simulink model "generator_simulink"  (R2022a)
settings: Solver=VariableStepAuto  StartTime=0.1  StopTime=90  FixedStep=sample_time/10  RelTol=1e-3
values from neighbouring files (symbols this model uses):
  B_eq = rotor.B + generator.B/gearbox.ratio^2    [parameters.m]
  G_noR = Yq*Gc    [generator_m.m]
  Gc = 1/(1 + s*tau_c)    [generator_m.m]    (also in generator_test.m)
  I_eq = rotor.I/gearbox.ratio^2 + generator.I    [main.m]    (also in parameters.m = rotor.I + generator.I/gearbox.ratio^2)
  Iq_ref = 12e3    (= 12000)    [generator_m.m]    (also in generator_test.m = 5000)
  Mr = 1e5    (= 100000)    [generator_m.m]    (also in generator_test.m)
  omega_r_ref = 1    [generator_m.m]    (also in generator_test.m)
  Riq = kiq_p + 1/s*kiq_i + s*kiq_d    [generator_m.m]    (also in generator_test.m)
  Riq_den = Riq.den{1}    [generator_m.m]
  Riq_num = Riq.num{1}    [generator_m.m]
  Romega = komega_p + 1/s*komega_i + s*komega_d    [generator_test.m]
  Yiq = (B+s*I)/(L*I*s^2+(R*I+L*B)*s+R*B+1.5*(p*Lambda)^2)    [generator_test.m]
  Yq = (B + s*I)/(1.5*(p*Lambda)^2*(1 + 2/3*(R + s*L)*(B + s*I)    /(p*Lambda)^2))    [generator_m.m]
undefined symbols (not defined in the file or in its folder): gearbox, generator, omega_r, R_omega_den, R_omega_num, rotor
settings Model: Creator=Niccolò  LastModifiedBy=Niccolò

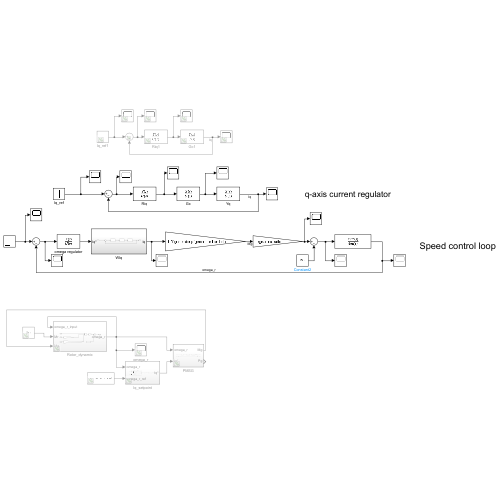
[thumbnail: Simulink's stored preview of the top-level diagram]
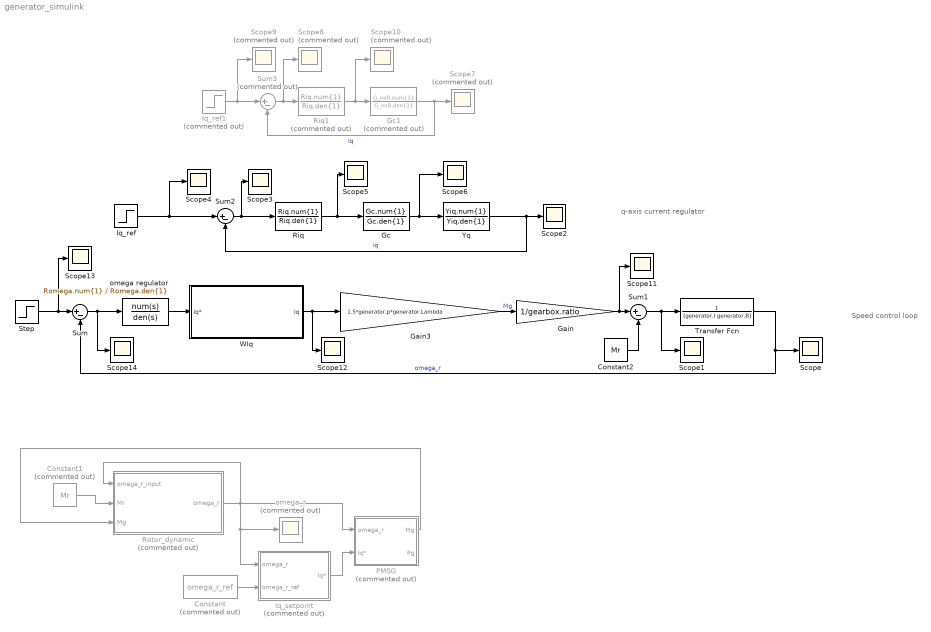
== system generator_simulink ==
  note: Speed control loop
  note: q-axis current regulator
  Constant : Constant  Commented=on  Value=omega_r_ref
  Constant1 : Constant  Commented=on  Value=Mr
  Constant2 : Constant  Value=Mr
  Gain : Gain  Gain=1/gearbox.ratio
  Gain3 : Gain  Gain=1.5*generator.p*generator.Lambda
  Gc : TransferFcn  Numerator=Gc.num{1}  Denominator=Gc.den{1}
  Gc1 : TransferFcn  Commented=on  Numerator=G_noR.num{1}  Denominator=G_noR.den{1}
  Iq_ref : Step  After=Iq_ref  SampleTime=0
  Iq_ref1 : Step  Commented=on  After=Iq_ref  SampleTime=0
  Iq_setpoint : Subsystem  Commented=on
  PMSG : Subsystem  Commented=on
  Riq : TransferFcn  Numerator=Riq.num{1}  Denominator=Riq.den{1}
  Riq1 : TransferFcn  Commented=on  Numerator=Riq.num{1}  Denominator=Riq.den{1}
  Rotor_dynamic : Subsystem  Commented=on
  Scope{,1..6,11..14} (11 alike) : Scope
  Scope{7..10} (4 alike) : Scope  Commented=on
  Step : Step  After=omega_r_ref  SampleTime=0
  Sum : Sum  Inputs=|+-
  Sum1 : Sum  Inputs=|+-
  Sum2 : Sum  Inputs=|+-
  Sum3 : Sum  Commented=on  Inputs=|+-
  Transfer Fcn : TransferFcn  Denominator=[generator.I generator.B]
  WIq : Subsystem
  Yq : TransferFcn  Numerator=Yiq.num{1}  Denominator=Yiq.den{1}
  omega regulator : TransferFcn  Numerator=Romega.num{1}  Denominator=Romega.den{1}
  omega_r : Scope  Commented=on
  wires:
  PMSG/1(Mg) -> Rotor_dynamic/3(Mg)
  Iq_setpoint/1(Iq*) -> PMSG/2(Iq*)
  Rotor_dynamic/1(omega_r) -> Iq_setpoint/1(omega_r), omega_r/1, PMSG/1(omega_r), Rotor_dynamic/1(omega_r_input)
  Constant/1 -> Iq_setpoint/2(omega_r_ref)
  Constant1/1 -> Rotor_dynamic/2(Mr)
  Gain3/1 -> Gain/1  "Mg"
  WIq/1(Iq) -> Scope12/1, Gain3/1
  Sum/1 -> Scope14/1, omega regulator/1
  Sum1/1 -> Scope1/1, Transfer Fcn/1
  Transfer Fcn/1 -> Scope/1, Sum/2  "omega_r"
  Constant2/1 -> Sum1/2
  Step/1 -> Scope13/1, Sum/1
  Riq/1 -> Scope5/1, Gc/1
  Gc/1 -> Scope6/1, Yq/1
  Sum2/1 -> Scope3/1, Riq/1
  Iq_ref/1 -> Scope4/1, Sum2/1
  Yq/1 -> Scope2/1, Sum2/2  "Iq"
  Riq1/1 -> Gc1/1, Scope10/1
  Gc1/1 -> Sum3/2, Scope7/1  "Iq"
  Sum3/1 -> Scope8/1, Riq1/1
  Iq_ref1/1 -> Scope9/1, Sum3/1
  omega regulator/1 -> WIq/1(Iq*)
  Gain/1 -> Scope11/1, Sum1/1

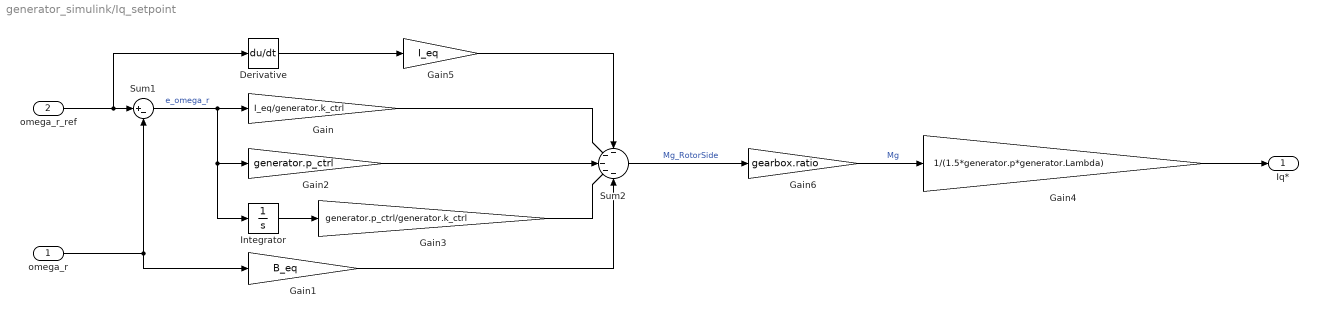
== system generator_simulink/Iq_setpoint ==
  omega_r : Inport
  omega_r_ref : Inport  Port=2
  Derivative : Derivative
  Gain : Gain  Gain=I_eq/generator.k_ctrl
  Gain1 : Gain  Gain=B_eq
  Gain2 : Gain  Gain=generator.p_ctrl
  Gain3 : Gain  Gain=generator.p_ctrl/generator.k_ctrl
  Gain4 : Gain  Gain=1/(1.5*generator.p*generator.Lambda)
  Gain5 : Gain  Gain=I_eq
  Gain6 : Gain  Gain=gearbox.ratio
  Integrator : Integrator
  Sum1 : Sum  Inputs=|+-
  Sum2 : Sum  Inputs=-----
  Iq* : Outport
  wires:
  Gain/1 -> Sum2/2
  Sum1/1 -> Integrator/1, Gain2/1, Gain/1  "e_omega_r"
  Gain1/1 -> Sum2/5
  Gain4/1 -> Iq*/1
  omega_r_ref/1 -> Derivative/1, Sum1/1
  omega_r/1 -> Gain1/1, Sum1/2
  Integrator/1 -> Gain3/1
  Gain3/1 -> Sum2/4
  Gain2/1 -> Sum2/3
  Sum2/1 -> Gain6/1  "Mg_RotorSide"
  Gain5/1 -> Sum2/1
  Gain6/1 -> Gain4/1  "Mg"
  Derivative/1 -> Gain5/1

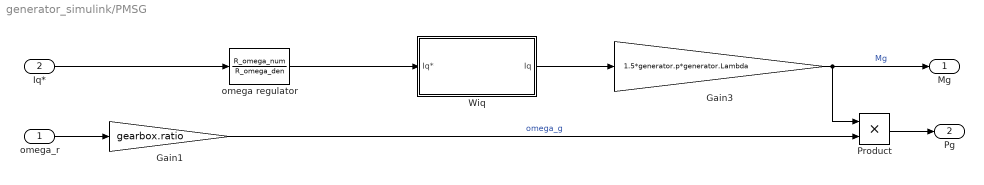
== system generator_simulink/PMSG ==
  omega_r : Inport
  Iq* : Inport  Port=2
  Gain1 : Gain  Gain=gearbox.ratio
  Gain3 : Gain  Gain=1.5*generator.p*generator.Lambda
  Product : Product
  Wiq : Subsystem
  omega regulator : TransferFcn  Numerator=R_omega_num  Denominator=R_omega_den
  Mg : Outport
  Pg : Outport  Port=2
  wires:
  omega_r/1 -> Gain1/1
  Gain3/1 -> Product/1, Mg/1  "Mg"
  Gain1/1 -> Product/2  "omega_g"
  Product/1 -> Pg/1
  Iq*/1 -> omega regulator/1
  Wiq/1(Iq) -> Gain3/1
  omega regulator/1 -> Wiq/1(Iq*)

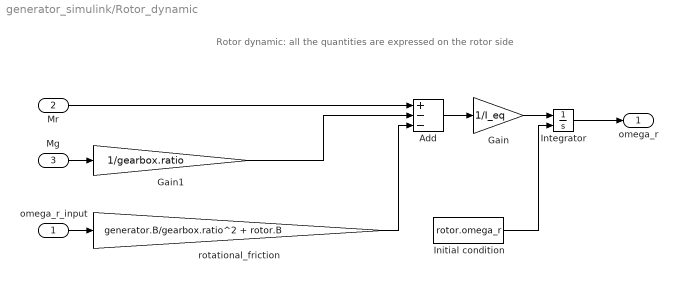
== system generator_simulink/Rotor_dynamic ==
  note: Rotor dynamic: all the quantities are expressed on the rotor side
  omega_r_input : Inport
  Mr : Inport  Port=2
  Mg : Inport  Port=3
  Add : Sum  Inputs=+--
  Gain : Gain  Gain=1/I_eq
  Gain1 : Gain  Gain=1/gearbox.ratio
  Initial condition : Constant  Value=rotor.omega_r
  Integrator : Integrator  InitialConditionSource=external  InitialCondition=omega_r
  rotational_friction : Gain  Gain=generator.B/gearbox.ratio^2 + rotor.B
  omega_r : Outport
  wires:
  Add/1 -> Gain/1
  Gain/1 -> Integrator/1
  Mr/1 -> Add/1
  Initial condition/1 -> Integrator/2
  omega_r_input/1 -> rotational_friction/1
  rotational_friction/1 -> Add/3
  Mg/1 -> Gain1/1
  Gain1/1 -> Add/2
  Integrator/1 -> omega_r/1

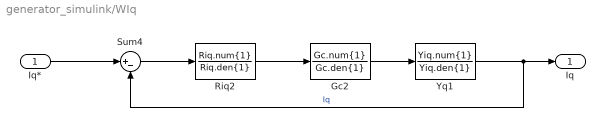
== system generator_simulink/WIq ==
  Iq* : Inport
  Gc2 : TransferFcn  Numerator=Gc.num{1}  Denominator=Gc.den{1}
  Riq2 : TransferFcn  Numerator=Riq.num{1}  Denominator=Riq.den{1}
  Sum4 : Sum  Inputs=|+-
  Yq1 : TransferFcn  Numerator=Yiq.num{1}  Denominator=Yiq.den{1}
  Iq : Outport
  wires:
  Yq1/1 -> Iq/1, Sum4/2  "Iq"
  Sum4/1 -> Riq2/1
  Riq2/1 -> Gc2/1
  Iq*/1 -> Sum4/1
  Gc2/1 -> Yq1/1

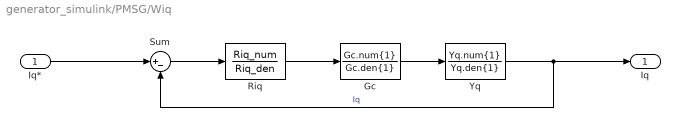
== system generator_simulink/PMSG/Wiq ==
  Iq* : Inport
  Gc : TransferFcn  Numerator=Gc.num{1}  Denominator=Gc.den{1}
  Riq : TransferFcn  Numerator=Riq_num  Denominator=Riq_den
  Sum : Sum  Inputs=|+-
  Yq : TransferFcn  Numerator=Yq.num{1}  Denominator=Yq.den{1}
  Iq : Outport
  wires:
  Riq/1 -> Gc/1
  Yq/1 -> Iq/1, Sum/2  "Iq"
  Sum/1 -> Riq/1
  Gc/1 -> Yq/1
  Iq*/1 -> Sum/1
